simulink model "steppidsupport"  (Simulink 5.0)
settings: Solver=ode45  StartTime=0.0  StopTime=29.9132  FixedStep=0.005  RelTol=1e-5
settings Model: Creator=root  LastModifiedBy=william  SaveTime=off  SaveOutput=off  RTWOptions="-aEnforceIntegerDowncast=1 -aExtMode=0 -aExtModeTesting=0 -aFoldNonRolledExpr=1 -aForceParamTrailComments=0 -aGenerateComments=1 -aGenerateReport=0 -aIgnoreCustomStorageClasses=1 -aIncDataTypeInIds=0 -aIncHierarchyInIds=0 -aInlineInvariantSignals=0 -aInlinedPrmAccess=\"Literals\" -aLocalBlockOutputs=1 -aLogVarNameModifier=\"rt_\" -aMaxRTWIdLen=31 -aPrefixModelToSubsysFcnNames=1 -aRTWVerbose=1 -aRollThreshold=5 -aShowEliminatedStatements=0"

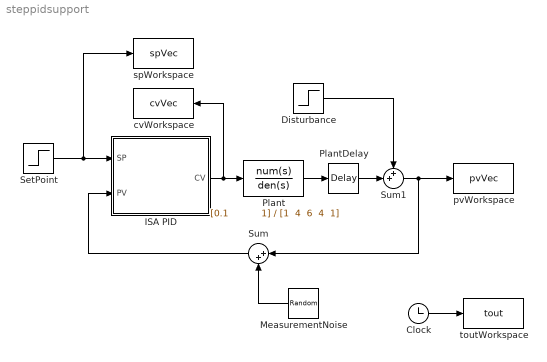
== system steppidsupport ==
  Clock : Clock
      settings: Decimation=10
  Disturbance : Step  Time=19.9422  After=0.1  SampleTime=0
  ISA PID : Subsystem  mask{uaw=[-5 5], Ts=0.019995, As=1, histLevel=0}
      mask prompts: uaw "Antiwindup saturation ([umin,umax])"; Ts "Sample time (Ts)"; As "Amplitude of the identifcation step or relay (A)"; histLevel "Histeresys of the relay"
      mask init:
      | umin = uaw(1);
      | umax = uaw(2);
      mask Display: disp('ISA PID')
  MeasurementNoise : RandomNumber  Orientation=left  Variance=0  SampleTime=0
  Plant : TransferFcn  Numerator="[0.1           1]"  Denominator="[1  4  6  4  1]"
  PlantDelay : TransportDelay  DelayTime=0.75
  SetPoint : Step  Time=0  SampleTime=0
  Sum : Sum  Orientation=left  Inputs=|++  SaturateOnIntegerOverflow=on  InputSameDT=on
  Sum1 : Sum  Inputs=++|  SaturateOnIntegerOverflow=on  InputSameDT=on
  cvWorkspace : ToWorkspace  VariableName=cvVec  SampleTime=0.019995  SaveFormat=Array
  pvWorkspace : ToWorkspace  VariableName=pvVec  SampleTime=0.019995  SaveFormat=Array
  spWorkspace : ToWorkspace  VariableName=spVec  SampleTime=0.019995  SaveFormat=Array
  toutWorkspace : ToWorkspace  VariableName=tout  SampleTime=0.019995  SaveFormat=Array
  wires:
  SetPoint/1 -> spWorkspace/1, ISA PID/1(SP)
  ISA PID/1(CV) -> cvWorkspace/1, Plant/1
  MeasurementNoise/1 -> Sum/2
  Sum/1 -> ISA PID/2(PV)
  Clock/1 -> toutWorkspace/1
  Sum1/1 -> pvWorkspace/1, Sum/1
  Disturbance/1 -> Sum1/1
  Plant/1 -> PlantDelay/1
  PlantDelay/1 -> Sum1/2

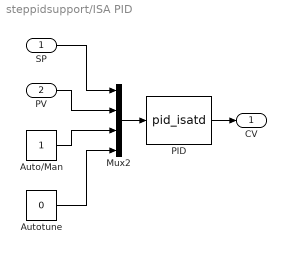
== system steppidsupport/ISA PID ==
  SP : Inport
  PV : Inport  Port=2
  Auto/Man : Constant
  Autotune : Constant  Value=0
  Mux2 : Mux
  PID : S-Function  FunctionName=pid_isatd  Parameters=Ts,umin,umax,As,histLevel
  CV : Outport
  wires:
  SP/1 -> Mux2/1
  PV/1 -> Mux2/2
  PID/1 -> CV/1
  Mux2/1 -> PID/1
  Auto/Man/1 -> Mux2/3
  Autotune/1 -> Mux2/4
